simulink model "DLS_ex2"  (R2025b)
(part 2 of 17)

  L_B25/LConn1 -- Heat Flow Rate Sensor49/RConn1
  B25/RConn1 -- 1.5_PULLEY/LConn2
  L_B6/LConn1 -- Heat Flow Rate Sensor52/RConn1
  Heat Flow Rate Sensor52/LConn1 -- B6/LConn1
  Heat Flow Rate Sensor52/RConn2 -- 1.5_PULLEY/LConn4
  B6/RConn1 -- Temperature Source15/LConn1
  A38/LConn1 -- Temperature Sensor37/LConn1 -- 4.7_TI_FLEXURE/RConn1
  Heat Flow Rate Sensor25/RConn2 -- A38/RConn1
  Temperature Sensor37/RConn2 -- T_A38/LConn1
  Thermal Reference37/LConn1 -- Temperature Sensor37/RConn1
  Simulink-PS Converter18/RConn1 -- A38/LConn2
  Heat Flow Rate Sensor25/RConn1 -- L_A38/LConn1
  Heat Flow Rate Sensor25/LConn1 -- 3.1_SMARACT_STAGE_ROTARY/LConn3
  L_A26/LConn1 -- 2.5_BRAID_ASSEMBLY/LConn2
  L_A27/LConn1 -- 2.5_BRAID_ASSEMBLY/LConn3
  L_A23/LConn1 -- 2.3_BRAID_ASSEMBLY/LConn5
  L_A22/LConn1 -- 2.3_BRAID_ASSEMBLY/LConn3
  4.7_TI_FLEXURE/RConn2 -- T_4.7.1X/LConn1
  4.7_TI_FLEXURE/RConn3 -- T_4.7.1/LConn1
  4.7_TI_FLEXURE/RConn4 -- T_4.7.12/LConn1
  4.7_TI_FLEXURE/RConn5 -- T_4.7.2/LConn1
  4.7_TI_FLEXURE/RConn6 -- T_4.7.234/LConn1
  4.7_TI_FLEXURE/RConn7 -- T_4.7.3/LConn1
  4.7_TI_FLEXURE/RConn8 -- T_4.7.4/LConn1
  4.7_TI_FLEXURE/RConn9 -- T_4.7.45/LConn1
  4.7_TI_FLEXURE/RConn10 -- T_4.7.5/LConn1
  4.7_TI_FLEXURE/RConn11 -- T_4.7.56/LConn1
  4.7_TI_FLEXURE/RConn12 -- T_4.7.6/LConn1
  4.7_TI_FLEXURE/RConn13 -- T_4.7.6X/LConn1
  HEATER_3/RConn1 -- 4.4_INSULATOR/LConn2
  T_INS/LConn1 -- 4.4_INSULATOR/LConn3
  Heat Flow Rate Sensor53/LConn1 -- B26/LConn1
  L_B26/LConn1 -- Heat Flow Rate Sensor53/RConn1
  Heat Flow Rate Sensor53/RConn2 -- 7.1 CABLE ASSEMBLY/RConn4
  Temperature Source14/LConn1 -- B26/RConn1
  Heat Flow Rate Sensor54/LConn1 -- B27/LConn1
  Heat Flow Rate Sensor54/RConn2 -- 7.1 CABLE ASSEMBLY/RConn3
  L_B27/LConn1 -- Heat Flow Rate Sensor54/RConn1
  B27/RConn1 -- 3.1_SMARACT_STAGE_ROTARY/LConn4
  Temperature Sensor38/LConn1 -- 4.7_TI_FLEXURE1/RConn1 -- A2/LConn1
  Heat Flow Rate Sensor55/LConn1 -- 3.1_SMARACT_STAGE_ROTARY/LConn2
  Thermal Reference38/LConn1 -- Temperature Sensor38/RConn1
  Heat Flow Rate Sensor55/RConn1 -- L_A29/LConn1
  Heat Flow Rate Sensor55/RConn2 -- A2/RConn1
  Temperature Sensor38/RConn2 -- T_A2/LConn1
  Simulink-PS Converter19/RConn1 -- A2/LConn2
  A37.4/LConn1 -- 4.7_TI_FLEXURE1/LConn5 -- Temperature Sensor39/LConn1
  A37.5/LConn1 -- Temperature Sensor40/LConn1 -- 4.7_TI_FLEXURE1/LConn6
  A37.6/LConn1 -- Temperature Sensor41/LConn1 -- 4.7_TI_FLEXURE1/LConn7
  Heat Flow Rate Sensor57/LConn1 -- 2.6_RIGID_SHIELD/RConn5
  Thermal Reference40/LConn1 -- Temperature Sensor40/RConn1
  Temperature Sensor40/RConn2 -- T_A37.5/LConn1
  Heat Flow Rate Sensor56/RConn2 -- A37.6/RConn1
  Thermal Reference41/LConn1 -- Temperature Sensor41/RConn1
  Heat Flow Rate Sensor56/LConn1 -- 2.6_RIGID_SHIELD/RConn3
  L_A37.5/LConn1 -- Heat Flow Rate Sensor58/RConn1
  Simulink-PS Converter20/RConn1 -- A37.4/LConn2
  Temperature Sensor39/RConn2 -- T_A37.4/LConn1
  Simulink-PS Converter21/RConn1 -- A37.5/LConn2
  Thermal Reference39/LConn1 -- Temperature Sensor39/RConn1
  Heat Flow Rate Sensor58/RConn2 -- A37.5/RConn1
  L_A37.4/LConn1 -- Heat Flow Rate Sensor57/RConn1
  Temperature Sensor41/RConn2 -- T_A37.6/LConn1
  L_A37.6/LConn1 -- Heat Flow Rate Sensor56/RConn1
  Heat Flow Rate Sensor57/RConn2 -- A37.4/RConn1
  Heat Flow Rate Sensor58/LConn1 -- 2.6_RIGID_SHIELD/RConn4
  Simulink-PS Converter22/RConn1 -- A37.6/LConn2
